simulink library "Testrig_4Post_Inputs"  (R2026a)
settings: Solver=VariableStepAuto
undefined symbols (not defined in the file or in its folder): Maneuver
libraries: dspsrcs4 x31, $bdroot x10, simulink x2
Description:
  | Testrig Inputs 4-Post Testrig
  | 
  | Copyright 2018-2024 The MathWorks, Inc.
settings Model: Creator=smiller  LastModifiedBy=andrei

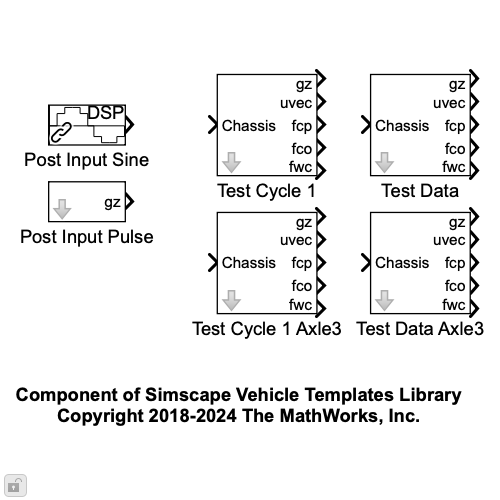
[thumbnail: Simulink's stored preview of the top-level diagram]
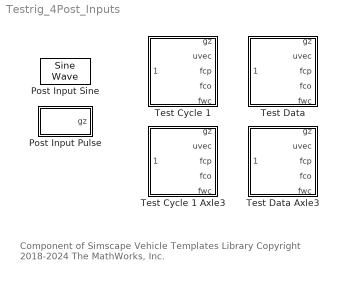
== system Testrig_4Post_Inputs ==
  note: Component of Simscape Vehicle Templates Library
      | Copyright 2018-2024 The MathWorks, Inc.
  Post Input Pulse : Subsystem  mask(Smooth Pulse){rise_time=0.1, pulse_length=2, wave_amplitude=5, wave_delay=1}
      mask prompts: rise_time "Rise/Fall Time (sec)"; pulse_length "Pulse Length (sec)"; wave_amplitude "Amplitude (m)"; wave_delay "Delay (sec)"
      mask help: Produces a pulse with a smooth start and finish, starting at a chosen time.
  Post Input Sine : dspsrcs4/Sine Wave  Amplitude=1  Frequency=100  Phase=0  SampleMode=Discrete  OutComplex=Real  CompMethod=Trigonometric fcn  TableSize=Speed  SampleTime=1/1000  SamplesPerFrame=1  ResetState=Restart at time zero  OutputFrames=off  dataType=double  wordLen=16  udDataType=sfix(16)  fracBitsMode=Best precision  numFracBits=15  OutDataTypeStr=double  LastOutDataTypeStr=double
  Test Cycle 1 : Subsystem  VariantControl=Test_Cycle_1  mask(Time-Based Post Height, Test Cycle 1, Four Posts){}
      mask help:
      | Sets road height beneath wheels to simulate a set of four tests: pitch, heave, roll, and bump.  The first three tests are sinusoidal, the last test is a trapezoid.
      |
      | This test is parameterized using the Maneuver data structure.  Use function sm_car_maneuverdata_testrig4Post_cycle1.m to create Maneuver and define this test.
  Test Cycle 1 Axle3 : Subsystem  mask(Time-Based Post Height, Test Cycle 1, 6 Posts){}
      mask help:
      | Sets road height beneath wheels to simulate a set of four tests: pitch, heave, roll, and bump.  The first three tests are sinusoidal, the last test is a trapezoid.
      |
      | This test is parameterized using the Maneuver data structure.  Use function sm_car_maneuverdata_testrig4Post_cycle1.m to create Maneuver and define this test.
  Test Data : Subsystem  VariantControl=Test_Cycle_1  mask(Time-Based Road Height, Four Post){table_postL1=Maneuver.PostL1.z.Value, brkpts_postL1=Maneuver.PostL1.t.Value, interp_postL1=Maneuver.PostL1.InterpMethod.Value, table_postR1=Maneuver.PostR1.z.Value, brkpts_postR1=Maneuver.PostR1.t.Value, interp_postR1=Maneuver.PostR1.InterpMethod.Value, table_postL2=Maneuver.PostL2.z.Value, brkpts_postL2=Maneuver.PostL2.t.Value, interp_postL2=Maneuver.PostL2.InterpMethod.Value, table_postR2=Maneuver.PostR2.z.Value, brkpts_postR2=Maneuver.PostR2.t.Value, interp_postR2=Maneuver.PostR2.InterpMethod.Value}
      mask prompts: table_postL1 "Height (m)"; brkpts_postL1 "Time (sec)"; interp_postL1 "Interpolation"; table_postR1 "Height (m)"; brkpts_postR1 "Time (sec)"; interp_postR1 "Interpolation"; table_postL2 "Height (m)"; brkpts_postL2 "Time (sec)"; interp_postL2 "Interpolation"; table_postR2 "Height (m)"; brkpts_postR2 "Time (sec)"; interp_postR2 "Interpolation"
      mask help: Sets road height based on simulation time. Used in postrig tests to control post based on generated or measured data. Set interpolation method to a string value that matches options for Lookup Table 1D block. Other outputs are held at their defaults.
      mask init:
      | bh = gcb;
      | set_param([bh '/Lookup Table L1'],'InterpMethod',interp_postL1);
      | set_param([bh '/Lookup Table R1'],'InterpMethod',interp_postR1);
      | set_param([bh '/Lookup Table L2'],'InterpMethod',interp_postL2);
      | set_param([bh '/Lookup Table R2'],'InterpMethod',interp_postR2);
      mask TypeOptions table_postL1: Lookup Table L1/Table
      mask TypeOptions brkpts_postL1: Lookup Table L1/BreakpointsForDimension1
      mask TypeOptions table_postR1: Lookup Table R1/Table
      mask TypeOptions brkpts_postR1: Lookup Table R1/BreakpointsForDimension1
      mask TypeOptions table_postL2: Lookup Table L2/Table
      mask TypeOptions brkpts_postL2: Lookup Table L2/BreakpointsForDimension1
      mask TypeOptions table_postR2: Lookup Table R2/Table
      mask TypeOptions brkpts_postR2: Lookup Table R2/BreakpointsForDimension1
      mask DialogControl cont_postL1 Prompt: Post L1 (Front Left)
      mask DialogControl cont_postR1 Prompt: Post R1 (Front Right)
      mask DialogControl cont_postL2 Prompt: Post L2 (Rear Left)
      mask DialogControl cont_postR2 Prompt: Post R2 (Rear Right)
  Test Data Axle3 : Subsystem  VariantControl=Test_Cycle_1  mask(Time-Based Road Height, Six Post Testrig){table_postL1=Maneuver.PostL1.z.Value, brkpts_postL1=Maneuver.PostL1.t.Value, interp_postL1=Maneuver.PostL1.InterpMethod.Value, table_postR1=Maneuver.PostR1.z.Value, brkpts_postR1=Maneuver.PostR1.t.Value, interp_postR1=Maneuver.PostR1.InterpMethod.Value, table_postL2=Maneuver.PostL2.z.Value, brkpts_postL2=Maneuver.PostL2.t.Value, interp_postL2=Maneuver.PostL2.InterpMethod.Value, table_postR2=Maneuver.PostR2.z.Value, brkpts_postR2=Maneuver.PostR2.t.Value, interp_postR2=Maneuver.PostR2.InterpMethod.Value, table_postL3=Maneuver.PostL3.z.Value, brkpts_postL3=Maneuver.PostL3.t.Value, interp_postL3=Maneuver.PostL3.InterpMethod.Value, table_postR3=Maneuver.PostR3.z.Value, brkpts_postR3=Maneuver.PostR3.t.Value, interp_postR3=Maneuver.PostR3.InterpMethod.Value}
      mask prompts: table_postL1 "Height (m)"; brkpts_postL1 "Time (sec)"; interp_postL1 "Interpolation"; table_postR1 "Height (m)"; brkpts_postR1 "Time (sec)"; interp_postR1 "Interpolation"; table_postL2 "Height (m)"; brkpts_postL2 "Time (sec)"; interp_postL2 "Interpolation"; table_postR2 "Height (m)"; brkpts_postR2 "Time (sec)"; interp_postR2 "Interpolation"; table_postL3 "Height (m)"; brkpts_postL3 "Time (sec)"; interp_postL3 "Interpolation"; table_postR3 "Height (m)"; brkpts_postR3 "Time (sec)"; interp_postR3 "Interpolation"
      mask help: Sets road height based on simulation time. Used in six-post testrigs to control post height based on generated or measured data. Set interpolation method to a string value that matches options for Lookup Table 1D block. Other outputs are held at their defaults.
      mask init:
      | bh = gcb;
      | set_param([bh '/Lookup Table L1'],'InterpMethod',interp_postL1);
      | set_param([bh '/Lookup Table R1'],'InterpMethod',interp_postR1);
      | set_param([bh '/Lookup Table L2'],'InterpMethod',interp_postL2);
      | set_param([bh '/Lookup Table R2'],'InterpMethod',interp_postR2);
      | set_param([bh '/Lookup Table L3'],'InterpMethod',interp_postL3);
      | set_param([bh '/Lookup Table R3'],'InterpMethod',interp_postR3);
      mask TypeOptions table_postL1: Lookup Table L1/Table
      mask TypeOptions brkpts_postL1: Lookup Table L1/BreakpointsForDimension1
      mask TypeOptions table_postR1: Lookup Table R1/Table
      mask TypeOptions brkpts_postR1: Lookup Table R1/BreakpointsForDimension1
      mask TypeOptions table_postL2: Lookup Table L2/Table
      mask TypeOptions brkpts_postL2: Lookup Table L2/BreakpointsForDimension1
      mask TypeOptions table_postR2: Lookup Table R2/Table
      mask TypeOptions brkpts_postR2: Lookup Table R2/BreakpointsForDimension1
      mask TypeOptions table_postL3: Lookup Table L3/Table
      mask TypeOptions brkpts_postL3: Lookup Table L3/BreakpointsForDimension1
      mask TypeOptions table_postR3: Lookup Table R3/Table
      mask TypeOptions brkpts_postR3: Lookup Table R3/BreakpointsForDimension1
      mask DialogControl cont_postL1 Prompt: Post L1 (Axle 1, Left)
      mask DialogControl cont_postR1 Prompt: Post R1 (Axle 1, Right)
      mask DialogControl cont_postL2 Prompt: Post L2 (Axle 2, Left)
      mask DialogControl cont_postR2 Prompt: Post R2 (Axle 2, Right)
      mask DialogControl cont_postL3 Prompt: Post L3  (Axle 3, Left)
      mask DialogControl cont_postR3 Prompt: Post R3  (Axle 3, Right)

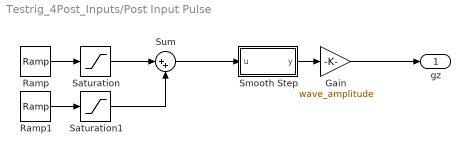
== system Testrig_4Post_Inputs/Post Input Pulse ==
  Gain : Gain  Gain=wave_amplitude
  Ramp : simulink/Sources/Ramp  slope=1/rise_time  start=wave_delay  InitialOutput=0
  Ramp1 : simulink/Sources/Ramp  slope=-1/rise_time  start=wave_delay+pulse_length-rise_time  InitialOutput=0
  Saturation : Saturate  UpperLimit=1  LowerLimit=0
  Saturation1 : Saturate  UpperLimit=0  LowerLimit=-1
  Smooth Step : Subsystem  mask(Smooth step function){step_start=0, step_finish=1, min_out=0, max_out=1}
      mask prompts: step_start "Start Step (u)"; step_finish "Finish Step (u)"; min_out "Minimum output (y)"; max_out "Maximum output (y)"
      mask help:
      | Smooth step function
      | y=3u^2-2u^3
      | Input and output ranges scaled by parameters.
  Sum : Sum  Inputs=|++
  gz : Outport  VectorParamsAs1DForOutWhenUnconnected=off
  wires:
  Gain/1 -> gz/1
  Ramp/1 -> Saturation/1
  Smooth Step/1(y) -> Gain/1
  Saturation/1 -> Sum/1
  Ramp1/1 -> Saturation1/1
  Saturation1/1 -> Sum/2
  Sum/1 -> Smooth Step/1(u)

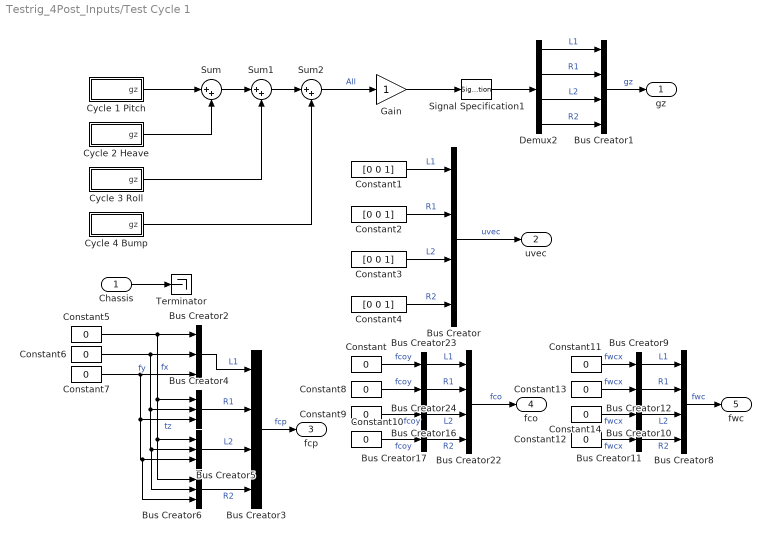
== system Testrig_4Post_Inputs/Test Cycle 1 ==
  Chassis : Inport
  Bus Creator{,1,3,8,22} (5 alike) : BusCreator  Inputs=4
  Bus Creator{9..12,16..17,23..24} (8 alike) : BusCreator  Inputs=1
  Bus Creator{2,4..6} (4 alike) : BusCreator  Inputs=3
  Constant{,5..14} (11 alike) : Constant  Value=0
  Constant{1..4} (4 alike) : Constant  Value=[0 0 1]
  Cycle 1 Pitch : Subsystem
  Cycle 2 Heave : Subsystem
  Cycle 3 Roll : Subsystem
  Cycle 4 Bump : Subsystem
  Demux2 : Demux
  Gain : Gain
  Signal Specification1 : SignalSpecification  Unit=m
  Sum : Sum  Inputs=|++
  Sum1 : Sum  Inputs=|++
  Sum2 : Sum  Inputs=|++
  Terminator : Terminator
  gz : Outport  VectorParamsAs1DForOutWhenUnconnected=off
  uvec : Outport  Port=2  VectorParamsAs1DForOutWhenUnconnected=off
  fcp : Outport  Port=3  VectorParamsAs1DForOutWhenUnconnected=off
  fco : Outport  Port=4  VectorParamsAs1DForOutWhenUnconnected=off
  fwc : Outport  Port=5  VectorParamsAs1DForOutWhenUnconnected=off
  wires:
  Constant7/1 -> Bus Creator2/3, Bus Creator4/3, Bus Creator5/3, Bus Creator6/3  "tz"
  Constant6/1 -> Bus Creator2/2, Bus Creator4/2, Bus Creator5/2, Bus Creator6/2  "fy"
  Constant5/1 -> Bus Creator2/1, Bus Creator4/1, Bus Creator5/1, Bus Creator6/1  "fx"
  Bus Creator6/1 -> Bus Creator3/4  "R2"
  Bus Creator5/1 -> Bus Creator3/3  "L2"
  Bus Creator2/1 -> Bus Creator3/1  "L1"
  Bus Creator4/1 -> Bus Creator3/2  "R1"
  Bus Creator3/1 -> fcp/1  "fcp"
  Cycle 2 Heave/1(gz) -> Sum/2
  Sum2/1 -> Gain/1  "All"
  Cycle 1 Pitch/1(gz) -> Sum/1
  Sum/1 -> Sum1/1
  Cycle 3 Roll/1(gz) -> Sum1/2
  Sum1/1 -> Sum2/1
  Cycle 4 Bump/1(gz) -> Sum2/2
  Gain/1 -> Signal Specification1/1
  Chassis/1 -> Terminator/1
  Constant4/1 -> Bus Creator/4  "R2"
  Bus Creator/1 -> uvec/1  "uvec"
  Constant1/1 -> Bus Creator/1  "L1"
  Constant2/1 -> Bus Creator/2  "R1"
  Constant3/1 -> Bus Creator/3  "L2"
  Signal Specification1/1 -> Demux2/1
  Demux2/3 -> Bus Creator1/3  "L2"
  Bus Creator1/1 -> gz/1  "gz"
  Demux2/4 -> Bus Creator1/4  "R2"
  Demux2/2 -> Bus Creator1/2  "R1"
  Demux2/1 -> Bus Creator1/1  "L1"
  Bus Creator12/1 -> Bus Creator8/2  "R1"
  Bus Creator24/1 -> Bus Creator22/2  "R1"
  Bus Creator10/1 -> Bus Creator8/3  "L2"
  Bus Creator9/1 -> Bus Creator8/1  "L1"
  Bus Creator16/1 -> Bus Creator22/3  "L2"
  Bus Creator22/1 -> fco/1  "fco"
  Bus Creator23/1 -> Bus Creator22/1  "L1"
  Bus Creator17/1 -> Bus Creator22/4  "R2"
  Constant8/1 -> Bus Creator24/1  "fcoy"
  Constant10/1 -> Bus Creator17/1  "fcoy"
  Constant9/1 -> Bus Creator16/1  "fcoy"
  Constant12/1 -> Bus Creator11/1  "fwcx"
  Constant14/1 -> Bus Creator10/1  "fwcx"
  Constant13/1 -> Bus Creator12/1  "fwcx"
  Bus Creator8/1 -> fwc/1  "fwc"
  Constant11/1 -> Bus Creator9/1  "fwcx"
  Constant/1 -> Bus Creator23/1  "fcoy"
  Bus Creator11/1 -> Bus Creator8/4  "R2"

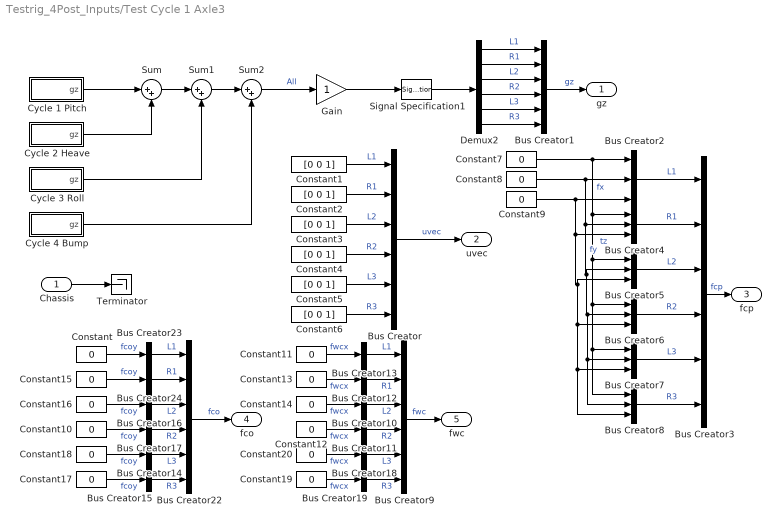
== system Testrig_4Post_Inputs/Test Cycle 1 Axle3 ==
  Chassis : Inport
  Bus Creator{,1,3,9,22} (5 alike) : BusCreator  Inputs=6
  Bus Creator{10..19,23..24} (12 alike) : BusCreator  Inputs=1
  Bus Creator{2,4..8} (6 alike) : BusCreator  Inputs=3
  Constant{,7..20} (15 alike) : Constant  Value=0
  Constant{1..6} (6 alike) : Constant  Value=[0 0 1]
  Cycle 1 Pitch : Subsystem
  Cycle 2 Heave : Subsystem
  Cycle 3 Roll : Subsystem
  Cycle 4 Bump : Subsystem
  Demux2 : Demux  Outputs=6
  Gain : Gain
  Signal Specification1 : SignalSpecification  Unit=m
  Sum : Sum  Inputs=|++
  Sum1 : Sum  Inputs=|++
  Sum2 : Sum  Inputs=|++
  Terminator : Terminator
  gz : Outport  VectorParamsAs1DForOutWhenUnconnected=off
  uvec : Outport  Port=2  VectorParamsAs1DForOutWhenUnconnected=off
  fcp : Outport  Port=3  VectorParamsAs1DForOutWhenUnconnected=off
  fco : Outport  Port=4  VectorParamsAs1DForOutWhenUnconnected=off
  fwc : Outport  Port=5  VectorParamsAs1DForOutWhenUnconnected=off
  wires:
  Demux2/1 -> Bus Creator1/1  "L1"
  Demux2/2 -> Bus Creator1/2  "R1"
  Demux2/4 -> Bus Creator1/4  "R2"
  Bus Creator1/1 -> gz/1  "gz"
  Demux2/3 -> Bus Creator1/3  "L2"
  Signal Specification1/1 -> Demux2/1
  Constant3/1 -> Bus Creator/3  "L2"
  Constant2/1 -> Bus Creator/2  "R1"
  Constant1/1 -> Bus Creator/1  "L1"
  Bus Creator/1 -> uvec/1  "uvec"
  Constant4/1 -> Bus Creator/4  "R2"
  Chassis/1 -> Terminator/1
  Gain/1 -> Signal Specification1/1
  Cycle 4 Bump/1(gz) -> Sum2/2
  Sum1/1 -> Sum2/1
  Cycle 3 Roll/1(gz) -> Sum1/2
  Sum/1 -> Sum1/1
  Cycle 1 Pitch/1(gz) -> Sum/1
  Sum2/1 -> Gain/1  "All"
  Cycle 2 Heave/1(gz) -> Sum/2
  Constant6/1 -> Bus Creator/6  "R3"
  Constant5/1 -> Bus Creator/5  "L3"
  Demux2/5 -> Bus Creator1/5  "L3"
  Demux2/6 -> Bus Creator1/6  "R3"
  Bus Creator6/1 -> Bus Creator3/4  "R2"
  Bus Creator4/1 -> Bus Creator3/2  "R1"
  Constant7/1 -> Bus Creator2/1, Bus Creator8/1, Bus Creator7/1, Bus Creator6/1, Bus Creator5/1, Bus Creator4/1  "fx"
  Bus Creator2/1 -> Bus Creator3/1  "L1"
  Bus Creator3/1 -> fcp/1  "fcp"
  Bus Creator5/1 -> Bus Creator3/3  "L2"
  Constant8/1 -> Bus Creator2/2, Bus Creator5/2, Bus Creator8/2, Bus Creator7/2, Bus Creator6/2, Bus Creator4/2  "fy"
  Constant9/1 -> Bus Creator2/3, Bus Creator5/3, Bus Creator6/3, Bus Creator8/3, Bus Creator7/3, Bus Creator4/3  "tz"
  Bus Creator7/1 -> Bus Creator3/5  "L3"
  Bus Creator8/1 -> Bus Creator3/6  "R3"
  Bus Creator12/1 -> Bus Creator9/2  "R1"
  Bus Creator24/1 -> Bus Creator22/2  "R1"
  Bus Creator10/1 -> Bus Creator9/3  "L2"
  Bus Creator13/1 -> Bus Creator9/1  "L1"
  Bus Creator16/1 -> Bus Creator22/3  "L2"
  Bus Creator22/1 -> fco/1  "fco"
  Bus Creator23/1 -> Bus Creator22/1  "L1"
  Bus Creator17/1 -> Bus Creator22/4  "R2"
  Constant15/1 -> Bus Creator24/1  "fcoy"
  Constant10/1 -> Bus Creator17/1  "fcoy"
  Constant16/1 -> Bus Creator16/1  "fcoy"
  Constant12/1 -> Bus Creator11/1  "fwcx"
  Constant14/1 -> Bus Creator10/1  "fwcx"
  Constant13/1 -> Bus Creator12/1  "fwcx"
  Bus Creator9/1 -> fwc/1  "fwc"
  Constant11/1 -> Bus Creator13/1  "fwcx"
  Constant/1 -> Bus Creator23/1  "fcoy"
  Bus Creator11/1 -> Bus Creator9/4  "R2"
  Constant18/1 -> Bus Creator14/1  "fcoy"
  Constant17/1 -> Bus Creator15/1  "fcoy"
  Bus Creator15/1 -> Bus Creator22/6  "R3"
  Bus Creator14/1 -> Bus Creator22/5  "L3"
  Bus Creator19/1 -> Bus Creator9/6  "R3"
  Constant20/1 -> Bus Creator18/1  "fwcx"
  Constant19/1 -> Bus Creator19/1  "fwcx"
  Bus Creator18/1 -> Bus Creator9/5  "L3"

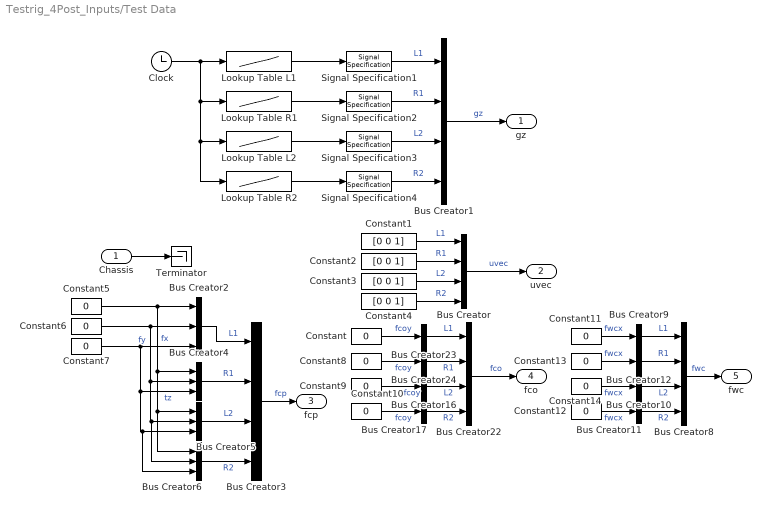
== system Testrig_4Post_Inputs/Test Data ==
  Chassis : Inport
  Bus Creator{,1,3,8,22} (5 alike) : BusCreator  Inputs=4
  Bus Creator{9..12,16..17,23..24} (8 alike) : BusCreator  Inputs=1
  Bus Creator{2,4..6} (4 alike) : BusCreator  Inputs=3
  Clock : Clock
  Constant{,5..14} (11 alike) : Constant  Value=0
  Constant{1..4} (4 alike) : Constant  Value=[0 0 1]
  Lookup Table L1 : Lookup_n-D  NumberOfTableDimensions=1  BreakpointsForDimension1=brkpts_postL1  Table=table_postL1  InternalRulePriority=Speed  RndMeth=Simplest
  Lookup Table L2 : Lookup_n-D  NumberOfTableDimensions=1  BreakpointsForDimension1=brkpts_postL2  Table=table_postL2  InterpMethod=Cubic spline  InternalRulePriority=Speed  RndMeth=Simplest
  Lookup Table R1 : Lookup_n-D  NumberOfTableDimensions=1  BreakpointsForDimension1=brkpts_postR1  Table=table_postR1  InterpMethod=Cubic spline  InternalRulePriority=Speed  RndMeth=Simplest
  Lookup Table R2 : Lookup_n-D  NumberOfTableDimensions=1  BreakpointsForDimension1=brkpts_postR2  Table=table_postR2  InterpMethod=Cubic spline  InternalRulePriority=Speed  RndMeth=Simplest
  Signal Specification{1..4} (4 alike) : SignalSpecification  Unit=m
  Terminator : Terminator
  gz : Outport  VectorParamsAs1DForOutWhenUnconnected=off
  uvec : Outport  Port=2  VectorParamsAs1DForOutWhenUnconnected=off
  fcp : Outport  Port=3  VectorParamsAs1DForOutWhenUnconnected=off
  fco : Outport  Port=4  VectorParamsAs1DForOutWhenUnconnected=off
  fwc : Outport  Port=5  VectorParamsAs1DForOutWhenUnconnected=off
  wires:
  Bus Creator11/1 -> Bus Creator8/4  "R2"
  Constant/1 -> Bus Creator23/1  "fcoy"
  Constant11/1 -> Bus Creator9/1  "fwcx"
  Bus Creator8/1 -> fwc/1  "fwc"
  Constant13/1 -> Bus Creator12/1  "fwcx"
  Constant14/1 -> Bus Creator10/1  "fwcx"
  Constant12/1 -> Bus Creator11/1  "fwcx"
  Constant9/1 -> Bus Creator16/1  "fcoy"
  Constant10/1 -> Bus Creator17/1  "fcoy"
  Constant8/1 -> Bus Creator24/1  "fcoy"
  Bus Creator17/1 -> Bus Creator22/4  "R2"
  Bus Creator23/1 -> Bus Creator22/1  "L1"
  Bus Creator22/1 -> fco/1  "fco"
  Bus Creator16/1 -> Bus Creator22/3  "L2"
  Bus Creator9/1 -> Bus Creator8/1  "L1"
  Bus Creator10/1 -> Bus Creator8/3  "L2"
  Bus Creator24/1 -> Bus Creator22/2  "R1"
  Bus Creator12/1 -> Bus Creator8/2  "R1"
  Constant3/1 -> Bus Creator/3  "L2"
  Constant2/1 -> Bus Creator/2  "R1"
  Constant1/1 -> Bus Creator/1  "L1"
  Bus Creator/1 -> uvec/1  "uvec"
  Constant4/1 -> Bus Creator/4  "R2"
  Chassis/1 -> Terminator/1
  Bus Creator3/1 -> fcp/1  "fcp"
  Bus Creator4/1 -> Bus Creator3/2  "R1"
  Bus Creator2/1 -> Bus Creator3/1  "L1"
  Bus Creator5/1 -> Bus Creator3/3  "L2"
  Bus Creator6/1 -> Bus Creator3/4  "R2"
  Constant5/1 -> Bus Creator6/1, Bus Creator5/1, Bus Creator4/1, Bus Creator2/1  "fx"
  Constant6/1 -> Bus Creator6/2, Bus Creator5/2, Bus Creator4/2, Bus Creator2/2  "fy"
  Constant7/1 -> Bus Creator6/3, Bus Creator5/3, Bus Creator4/3, Bus Creator2/3  "tz"
  Clock/1 -> Lookup Table L1/1, Lookup Table R2/1, Lookup Table L2/1, Lookup Table R1/1
  Lookup Table R2/1 -> Signal Specification4/1
  Bus Creator1/1 -> gz/1  "gz"
  Lookup Table L1/1 -> Signal Specification1/1
  Lookup Table L2/1 -> Signal Specification3/1
  Signal Specification3/1 -> Bus Creator1/3  "L2"
  Signal Specification2/1 -> Bus Creator1/2  "R1"
  Signal Specification1/1 -> Bus Creator1/1  "L1"
  Signal Specification4/1 -> Bus Creator1/4  "R2"
  Lookup Table R1/1 -> Signal Specification2/1

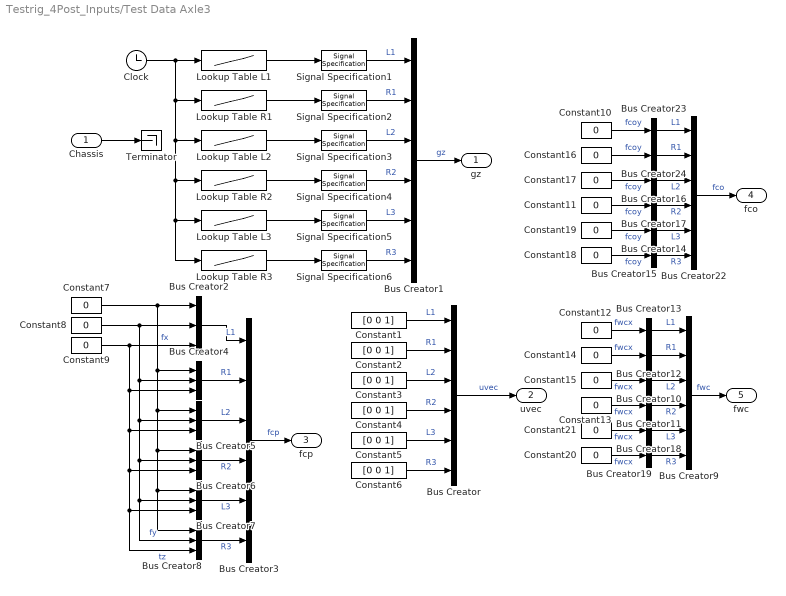
== system Testrig_4Post_Inputs/Test Data Axle3 ==
  Chassis : Inport
  Bus Creator{,1,3,9,22} (5 alike) : BusCreator  Inputs=6
  Bus Creator{10..19,23..24} (12 alike) : BusCreator  Inputs=1
  Bus Creator{2,4..8} (6 alike) : BusCreator  Inputs=3
  Clock : Clock
  Constant{1..6} (6 alike) : Constant  Value=[0 0 1]
  Constant{7..21} (15 alike) : Constant  Value=0
  Lookup Table L1 : Lookup_n-D  NumberOfTableDimensions=1  BreakpointsForDimension1=brkpts_postL1  Table=table_postL1  InternalRulePriority=Speed  RndMeth=Simplest
  Lookup Table L2 : Lookup_n-D  NumberOfTableDimensions=1  BreakpointsForDimension1=brkpts_postL2  Table=table_postL2  InterpMethod=Cubic spline  InternalRulePriority=Speed  RndMeth=Simplest
  Lookup Table L3 : Lookup_n-D  NumberOfTableDimensions=1  BreakpointsForDimension1=brkpts_postL3  Table=table_postL3  InterpMethod=Cubic spline  InternalRulePriority=Speed  RndMeth=Simplest
  Lookup Table R1 : Lookup_n-D  NumberOfTableDimensions=1  BreakpointsForDimension1=brkpts_postR1  Table=table_postR1  InterpMethod=Cubic spline  InternalRulePriority=Speed  RndMeth=Simplest
  Lookup Table R2 : Lookup_n-D  NumberOfTableDimensions=1  BreakpointsForDimension1=brkpts_postR2  Table=table_postR2  InterpMethod=Cubic spline  InternalRulePriority=Speed  RndMeth=Simplest
  Lookup Table R3 : Lookup_n-D  NumberOfTableDimensions=1  BreakpointsForDimension1=brkpts_postR3  Table=table_postR3  InterpMethod=Cubic spline  InternalRulePriority=Speed  RndMeth=Simplest
  Signal Specification{1..6} (6 alike) : SignalSpecification  Unit=m
  Terminator : Terminator
  gz : Outport  VectorParamsAs1DForOutWhenUnconnected=off
  uvec : Outport  Port=2  VectorParamsAs1DForOutWhenUnconnected=off
  fcp : Outport  Port=3  VectorParamsAs1DForOutWhenUnconnected=off
  fco : Outport  Port=4  VectorParamsAs1DForOutWhenUnconnected=off
  fwc : Outport  Port=5  VectorParamsAs1DForOutWhenUnconnected=off
  wires:
  Lookup Table R1/1 -> Signal Specification2/1
  Signal Specification4/1 -> Bus Creator1/4  "R2"
  Signal Specification1/1 -> Bus Creator1/1  "L1"
  Signal Specification2/1 -> Bus Creator1/2  "R1"
  Signal Specification3/1 -> Bus Creator1/3  "L2"
  Lookup Table L2/1 -> Signal Specification3/1
  Lookup Table L1/1 -> Signal Specification1/1
  Bus Creator1/1 -> gz/1  "gz"
  Lookup Table R2/1 -> Signal Specification4/1
  Chassis/1 -> Terminator/1
  Constant5/1 -> Bus Creator/5  "L3"
  Bus Creator2/1 -> Bus Creator3/1  "L1"
  Constant7/1 -> Bus Creator6/1, Bus Creator7/1, Bus Creator8/1, Bus Creator5/1, Bus Creator4/1, Bus Creator2/1  "fx"
  Constant6/1 -> Bus Creator/6  "R3"
  Bus Creator6/1 -> Bus Creator3/4  "R2"
  Constant18/1 -> Bus Creator15/1  "fcoy"
  Constant14/1 -> Bus Creator12/1  "fwcx"
  Bus Creator13/1 -> Bus Creator9/1  "L1"
  Constant17/1 -> Bus Creator16/1  "fcoy"
  Constant3/1 -> Bus Creator/3  "L2"
  Bus Creator19/1 -> Bus Creator9/6  "R3"
  Bus Creator4/1 -> Bus Creator3/2  "R1"
  Bus Creator22/1 -> fco/1  "fco"
  Bus Creator18/1 -> Bus Creator9/5  "L3"
  Bus Creator8/1 -> Bus Creator3/6  "R3"
  Bus Creator12/1 -> Bus Creator9/2  "R1"
  Constant2/1 -> Bus Creator/2  "R1"
  Bus Creator/1 -> uvec/1  "uvec"
  Bus Creator7/1 -> Bus Creator3/5  "L3"
  Constant4/1 -> Bus Creator/4  "R2"
  Bus Creator10/1 -> Bus Creator9/3  "L2"
  Constant11/1 -> Bus Creator17/1  "fcoy"
  Bus Creator14/1 -> Bus Creator22/5  "L3"
  Constant16/1 -> Bus Creator24/1  "fcoy"
  Constant12/1 -> Bus Creator13/1  "fwcx"
  Constant21/1 -> Bus Creator18/1  "fwcx"
  Constant1/1 -> Bus Creator/1  "L1"
  Constant10/1 -> Bus Creator23/1  "fcoy"
  Bus Creator11/1 -> Bus Creator9/4  "R2"
  Bus Creator23/1 -> Bus Creator22/1  "L1"
  Constant9/1 -> Bus Creator8/3, Bus Creator7/3, Bus Creator6/3, Bus Creator5/3, Bus Creator4/3, Bus Creator2/3  "tz"
  Bus Creator5/1 -> Bus Creator3/3  "L2"
  Constant15/1 -> Bus Creator10/1  "fwcx"
  Bus Creator15/1 -> Bus Creator22/6  "R3"
  Constant19/1 -> Bus Creator14/1  "fcoy"
  Constant13/1 -> Bus Creator11/1  "fwcx"
  Bus Creator3/1 -> fcp/1  "fcp"
  Bus Creator24/1 -> Bus Creator22/2  "R1"
  Constant8/1 -> Bus Creator8/2, Bus Creator7/2, Bus Creator6/2, Bus Creator5/2, Bus Creator4/2, Bus Creator2/2  "fy"
  Bus Creator16/1 -> Bus Creator22/3  "L2"
  Bus Creator17/1 -> Bus Creator22/4  "R2"
  Bus Creator9/1 -> fwc/1  "fwc"
  Constant20/1 -> Bus Creator19/1  "fwcx"
  Clock/1 -> Lookup Table R1/1, Lookup Table L2/1, Lookup Table R3/1, Lookup Table L3/1, Lookup Table R2/1, Lookup Table L1/1
  Lookup Table R3/1 -> Signal Specification6/1
  Lookup Table L3/1 -> Signal Specification5/1
  Signal Specification5/1 -> Bus Creator1/5  "L3"
  Signal Specification6/1 -> Bus Creator1/6  "R3"

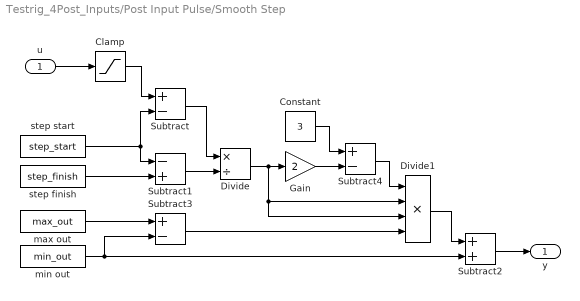
== system Testrig_4Post_Inputs/Post Input Pulse/Smooth Step ==
  u : Inport
  Clamp : Saturate  UpperLimit=step_finish  LowerLimit=step_start
  Constant : Constant  Value=3
  Divide : Product  Inputs=*/
  Divide1 : Product  Inputs=****
  Gain : Gain  Gain=2
  Subtract : Sum  Inputs=+-
  Subtract1 : Sum  Inputs=-+
  Subtract2 : Sum
  Subtract3 : Sum  Inputs=+-
  Subtract4 : Sum  Inputs=+-
  max out : Constant  Value=max_out
  min out : Constant  Value=min_out
  step finish : Constant  Value=step_finish
  step start : Constant  Value=step_start
  y : Outport  VectorParamsAs1DForOutWhenUnconnected=off
  wires:
  step start/1 -> Subtract1/1, Subtract/2
  u/1 -> Clamp/1
  Subtract1/1 -> Divide/2
  Divide/1 -> Gain/1, Divide1/2, Divide1/3
  Subtract/1 -> Divide/1
  Subtract2/1 -> y/1
  Constant/1 -> Subtract4/1
  min out/1 -> Subtract2/2, Subtract3/2
  max out/1 -> Subtract3/1
  Clamp/1 -> Subtract/1
  step finish/1 -> Subtract1/2
  Divide1/1 -> Subtract2/1
  Gain/1 -> Subtract4/2
  Subtract4/1 -> Divide1/1
  Subtract3/1 -> Divide1/4

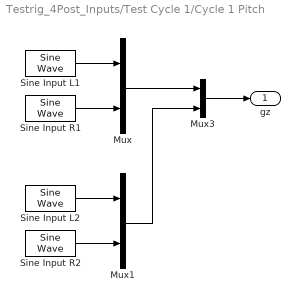
== system Testrig_4Post_Inputs/Test Cycle 1/Cycle 1 Pitch ==
  Mux : Mux  Inputs=2
  Mux1 : Mux  Inputs=2
  Mux3 : Mux  Inputs=2
  Sine Input L1 : dspsrcs4/Sine Wave  Amplitude=1  Frequency=100  Phase=0  SampleMode=Discrete  OutComplex=Real  CompMethod=Trigonometric fcn  TableSize=Speed  SampleTime=1/1000  SamplesPerFrame=1  ResetState=Restart at time zero  OutputFrames=off  dataType=double  wordLen=16  udDataType=sfix(16)  fracBitsMode=Best precision  numFracBits=15  OutDataTypeStr=double  LastOutDataTypeStr=double
  Sine Input L2 : dspsrcs4/Sine Wave  Amplitude=1  Frequency=100  Phase=0  SampleMode=Discrete  OutComplex=Real  CompMethod=Trigonometric fcn  TableSize=Speed  SampleTime=1/1000  SamplesPerFrame=1  ResetState=Restart at time zero  OutputFrames=off  dataType=double  wordLen=16  udDataType=sfix(16)  fracBitsMode=Best precision  numFracBits=15  OutDataTypeStr=double  LastOutDataTypeStr=double
  Sine Input R1 : dspsrcs4/Sine Wave  Amplitude=1  Frequency=100  Phase=0  SampleMode=Discrete  OutComplex=Real  CompMethod=Trigonometric fcn  TableSize=Speed  SampleTime=1/1000  SamplesPerFrame=1  ResetState=Restart at time zero  OutputFrames=off  dataType=double  wordLen=16  udDataType=sfix(16)  fracBitsMode=Best precision  numFracBits=15  OutDataTypeStr=double  LastOutDataTypeStr=double
  Sine Input R2 : dspsrcs4/Sine Wave  Amplitude=1  Frequency=100  Phase=0  SampleMode=Discrete  OutComplex=Real  CompMethod=Trigonometric fcn  TableSize=Speed  SampleTime=1/1000  SamplesPerFrame=1  ResetState=Restart at time zero  OutputFrames=off  dataType=double  wordLen=16  udDataType=sfix(16)  fracBitsMode=Best precision  numFracBits=15  OutDataTypeStr=double  LastOutDataTypeStr=double
  gz : Outport  VectorParamsAs1DForOutWhenUnconnected=off
  wires:
  Sine Input L1/1 -> Mux/1
  Sine Input R1/1 -> Mux/2
  Mux/1 -> Mux3/1
  Mux3/1 -> gz/1
  Mux1/1 -> Mux3/2
  Sine Input R2/1 -> Mux1/2
  Sine Input L2/1 -> Mux1/1

== system Testrig_4Post_Inputs/Test Cycle 1/Cycle 2 Heave ==
  Mux : Mux  Inputs=2
  Mux1 : Mux  Inputs=2
  Mux3 : Mux  Inputs=2
  Sine Input L1 : dspsrcs4/Sine Wave  Amplitude=1  Frequency=100  Phase=0  SampleMode=Discrete  OutComplex=Real  CompMethod=Trigonometric fcn  TableSize=Speed  SampleTime=1/1000  SamplesPerFrame=1  ResetState=Restart at time zero  OutputFrames=off  dataType=double  wordLen=16  udDataType=sfix(16)  fracBitsMode=Best precision  numFracBits=15  OutDataTypeStr=double  LastOutDataTypeStr=double
  Sine Input L2 : dspsrcs4/Sine Wave  Amplitude=1  Frequency=100  Phase=0  SampleMode=Discrete  OutComplex=Real  CompMethod=Trigonometric fcn  TableSize=Speed  SampleTime=1/1000  SamplesPerFrame=1  ResetState=Restart at time zero  OutputFrames=off  dataType=double  wordLen=16  udDataType=sfix(16)  fracBitsMode=Best precision  numFracBits=15  OutDataTypeStr=double  LastOutDataTypeStr=double
  Sine Input R1 : dspsrcs4/Sine Wave  Amplitude=1  Frequency=100  Phase=0  SampleMode=Discrete  OutComplex=Real  CompMethod=Trigonometric fcn  TableSize=Speed  SampleTime=1/1000  SamplesPerFrame=1  ResetState=Restart at time zero  OutputFrames=off  dataType=double  wordLen=16  udDataType=sfix(16)  fracBitsMode=Best precision  numFracBits=15  OutDataTypeStr=double  LastOutDataTypeStr=double
  Sine Input R2 : dspsrcs4/Sine Wave  Amplitude=1  Frequency=100  Phase=0  SampleMode=Discrete  OutComplex=Real  CompMethod=Trigonometric fcn  TableSize=Speed  SampleTime=1/1000  SamplesPerFrame=1  ResetState=Restart at time zero  OutputFrames=off  dataType=double  wordLen=16  udDataType=sfix(16)  fracBitsMode=Best precision  numFracBits=15  OutDataTypeStr=double  LastOutDataTypeStr=double
  gz : Outport  VectorParamsAs1DForOutWhenUnconnected=off
  wires:
  Sine Input L2/1 -> Mux1/1
  Sine Input R2/1 -> Mux1/2
  Mux1/1 -> Mux3/2
  Mux3/1 -> gz/1
  Mux/1 -> Mux3/1
  Sine Input R1/1 -> Mux/2
  Sine Input L1/1 -> Mux/1

== system Testrig_4Post_Inputs/Test Cycle 1/Cycle 3 Roll ==
  Mux : Mux  Inputs=2
  Mux1 : Mux  Inputs=2
  Mux3 : Mux  Inputs=2
  Sine Input L1 : dspsrcs4/Sine Wave  Amplitude=1  Frequency=100  Phase=0  SampleMode=Discrete  OutComplex=Real  CompMethod=Trigonometric fcn  TableSize=Speed  SampleTime=1/1000  SamplesPerFrame=1  ResetState=Restart at time zero  OutputFrames=off  dataType=double  wordLen=16  udDataType=sfix(16)  fracBitsMode=Best precision  numFracBits=15  OutDataTypeStr=double  LastOutDataTypeStr=double
  Sine Input L2 : dspsrcs4/Sine Wave  Amplitude=1  Frequency=100  Phase=0  SampleMode=Discrete  OutComplex=Real  CompMethod=Trigonometric fcn  TableSize=Speed  SampleTime=1/1000  SamplesPerFrame=1  ResetState=Restart at time zero  OutputFrames=off  dataType=double  wordLen=16  udDataType=sfix(16)  fracBitsMode=Best precision  numFracBits=15  OutDataTypeStr=double  LastOutDataTypeStr=double
  Sine Input R1 : dspsrcs4/Sine Wave  Amplitude=1  Frequency=100  Phase=0  SampleMode=Discrete  OutComplex=Real  CompMethod=Trigonometric fcn  TableSize=Speed  SampleTime=1/1000  SamplesPerFrame=1  ResetState=Restart at time zero  OutputFrames=off  dataType=double  wordLen=16  udDataType=sfix(16)  fracBitsMode=Best precision  numFracBits=15  OutDataTypeStr=double  LastOutDataTypeStr=double
  Sine Input R2 : dspsrcs4/Sine Wave  Amplitude=1  Frequency=100  Phase=0  SampleMode=Discrete  OutComplex=Real  CompMethod=Trigonometric fcn  TableSize=Speed  SampleTime=1/1000  SamplesPerFrame=1  ResetState=Restart at time zero  OutputFrames=off  dataType=double  wordLen=16  udDataType=sfix(16)  fracBitsMode=Best precision  numFracBits=15  OutDataTypeStr=double  LastOutDataTypeStr=double
  gz : Outport  VectorParamsAs1DForOutWhenUnconnected=off
  wires:
  Sine Input L1/1 -> Mux/1
  Sine Input R1/1 -> Mux/2
  Mux/1 -> Mux3/1
  Mux3/1 -> gz/1
  Mux1/1 -> Mux3/2
  Sine Input R2/1 -> Mux1/2
  Sine Input L2/1 -> Mux1/1

== system Testrig_4Post_Inputs/Test Cycle 1/Cycle 4 Bump ==
  Mux : Mux  Inputs=2
  Mux2 : Mux  Inputs=2
  Mux3 : Mux  Inputs=2
  Pulse Input L1 : $bdroot/Post Input Pulse  rise_time=Maneuver.Bump.L1.tRise.Value  pulse_length=Maneuver.Bump.L1.tDuration.Value  wave_amplitude=Maneuver.Bump.L1.xAmplitude.Value  wave_delay=Maneuver.Bump.L1.tStart.Value
  Pulse Input L2 : $bdroot/Post Input Pulse  rise_time=Maneuver.Bump.L2.tRise.Value  pulse_length=Maneuver.Bump.L2.tDuration.Value  wave_amplitude=Maneuver.Bump.L2.xAmplitude.Value  wave_delay=Maneuver.Bump.L2.tStart.Value
  Pulse Input R1 : $bdroot/Post Input Pulse  rise_time=Maneuver.Bump.R1.tRise.Value  pulse_length=Maneuver.Bump.R1.tDuration.Value  wave_amplitude=Maneuver.Bump.R1.xAmplitude.Value  wave_delay=Maneuver.Bump.R1.tStart.Value
  Pulse Input R2 : $bdroot/Post Input Pulse  rise_time=Maneuver.Bump.R2.tRise.Value  pulse_length=Maneuver.Bump.R2.tDuration.Value  wave_amplitude=Maneuver.Bump.R2.xAmplitude.Value  wave_delay=Maneuver.Bump.R2.tStart.Value
  gz : Outport  VectorParamsAs1DForOutWhenUnconnected=off
  wires:
  Mux2/1 -> Mux3/2
  Mux3/1 -> gz/1
  Mux/1 -> Mux3/1
  Pulse Input R2/1 -> Mux2/2
  Pulse Input R1/1 -> Mux/2
  Pulse Input L1/1 -> Mux/1
  Pulse Input L2/1 -> Mux2/1

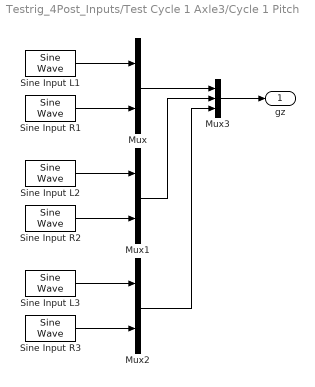
== system Testrig_4Post_Inputs/Test Cycle 1 Axle3/Cycle 1 Pitch ==
  Mux : Mux  Inputs=2
  Mux1 : Mux  Inputs=2
  Mux2 : Mux  Inputs=2
  Mux3 : Mux  Inputs=3
  Sine Input L1 : dspsrcs4/Sine Wave  Amplitude=1  Frequency=100  Phase=0  SampleMode=Discrete  OutComplex=Real  CompMethod=Trigonometric fcn  TableSize=Speed  SampleTime=1/1000  SamplesPerFrame=1  ResetState=Restart at time zero  OutputFrames=off  dataType=double  wordLen=16  udDataType=sfix(16)  fracBitsMode=Best precision  numFracBits=15  OutDataTypeStr=double  LastOutDataTypeStr=double
  Sine Input L2 : dspsrcs4/Sine Wave  Amplitude=1  Frequency=100  Phase=0  SampleMode=Discrete  OutComplex=Real  CompMethod=Trigonometric fcn  TableSize=Speed  SampleTime=1/1000  SamplesPerFrame=1  ResetState=Restart at time zero  OutputFrames=off  dataType=double  wordLen=16  udDataType=sfix(16)  fracBitsMode=Best precision  numFracBits=15  OutDataTypeStr=double  LastOutDataTypeStr=double
  Sine Input L3 : dspsrcs4/Sine Wave  Amplitude=1  Frequency=100  Phase=0  SampleMode=Discrete  OutComplex=Real  CompMethod=Trigonometric fcn  TableSize=Speed  SampleTime=1/1000  SamplesPerFrame=1  ResetState=Restart at time zero  OutputFrames=off  dataType=double  wordLen=16  udDataType=sfix(16)  fracBitsMode=Best precision  numFracBits=15  OutDataTypeStr=double  LastOutDataTypeStr=double
  Sine Input R1 : dspsrcs4/Sine Wave  Amplitude=1  Frequency=100  Phase=0  SampleMode=Discrete  OutComplex=Real  CompMethod=Trigonometric fcn  TableSize=Speed  SampleTime=1/1000  SamplesPerFrame=1  ResetState=Restart at time zero  OutputFrames=off  dataType=double  wordLen=16  udDataType=sfix(16)  fracBitsMode=Best precision  numFracBits=15  OutDataTypeStr=double  LastOutDataTypeStr=double
  Sine Input R2 : dspsrcs4/Sine Wave  Amplitude=1  Frequency=100  Phase=0  SampleMode=Discrete  OutComplex=Real  CompMethod=Trigonometric fcn  TableSize=Speed  SampleTime=1/1000  SamplesPerFrame=1  ResetState=Restart at time zero  OutputFrames=off  dataType=double  wordLen=16  udDataType=sfix(16)  fracBitsMode=Best precision  numFracBits=15  OutDataTypeStr=double  LastOutDataTypeStr=double
  Sine Input R3 : dspsrcs4/Sine Wave  Amplitude=1  Frequency=100  Phase=0  SampleMode=Discrete  OutComplex=Real  CompMethod=Trigonometric fcn  TableSize=Speed  SampleTime=1/1000  SamplesPerFrame=1  ResetState=Restart at time zero  OutputFrames=off  dataType=double  wordLen=16  udDataType=sfix(16)  fracBitsMode=Best precision  numFracBits=15  OutDataTypeStr=double  LastOutDataTypeStr=double
  gz : Outport  VectorParamsAs1DForOutWhenUnconnected=off
  wires:
  Sine Input L2/1 -> Mux1/1
  Sine Input R2/1 -> Mux1/2
  Mux1/1 -> Mux3/2
  Mux3/1 -> gz/1
  Mux/1 -> Mux3/1
  Sine Input R1/1 -> Mux/2
  Sine Input L1/1 -> Mux/1
  Mux2/1 -> Mux3/3
  Sine Input R3/1 -> Mux2/2
  Sine Input L3/1 -> Mux2/1

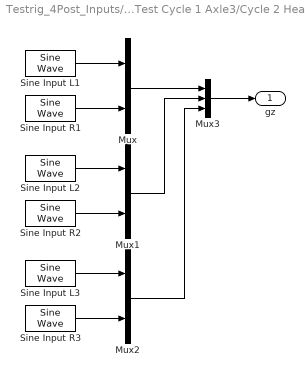
== system Testrig_4Post_Inputs/Test Cycle 1 Axle3/Cycle 2 Heave ==
  Mux : Mux  Inputs=2
  Mux1 : Mux  Inputs=2
  Mux2 : Mux  Inputs=2
  Mux3 : Mux  Inputs=3
  Sine Input L1 : dspsrcs4/Sine Wave  Amplitude=1  Frequency=100  Phase=0  SampleMode=Discrete  OutComplex=Real  CompMethod=Trigonometric fcn  TableSize=Speed  SampleTime=1/1000  SamplesPerFrame=1  ResetState=Restart at time zero  OutputFrames=off  dataType=double  wordLen=16  udDataType=sfix(16)  fracBitsMode=Best precision  numFracBits=15  OutDataTypeStr=double  LastOutDataTypeStr=double
  Sine Input L2 : dspsrcs4/Sine Wave  Amplitude=1  Frequency=100  Phase=0  SampleMode=Discrete  OutComplex=Real  CompMethod=Trigonometric fcn  TableSize=Speed  SampleTime=1/1000  SamplesPerFrame=1  ResetState=Restart at time zero  OutputFrames=off  dataType=double  wordLen=16  udDataType=sfix(16)  fracBitsMode=Best precision  numFracBits=15  OutDataTypeStr=double  LastOutDataTypeStr=double
  Sine Input L3 : dspsrcs4/Sine Wave  Amplitude=1  Frequency=100  Phase=0  SampleMode=Discrete  OutComplex=Real  CompMethod=Trigonometric fcn  TableSize=Speed  SampleTime=1/1000  SamplesPerFrame=1  ResetState=Restart at time zero  OutputFrames=off  dataType=double  wordLen=16  udDataType=sfix(16)  fracBitsMode=Best precision  numFracBits=15  OutDataTypeStr=double  LastOutDataTypeStr=double
  Sine Input R1 : dspsrcs4/Sine Wave  Amplitude=1  Frequency=100  Phase=0  SampleMode=Discrete  OutComplex=Real  CompMethod=Trigonometric fcn  TableSize=Speed  SampleTime=1/1000  SamplesPerFrame=1  ResetState=Restart at time zero  OutputFrames=off  dataType=double  wordLen=16  udDataType=sfix(16)  fracBitsMode=Best precision  numFracBits=15  OutDataTypeStr=double  LastOutDataTypeStr=double
  Sine Input R2 : dspsrcs4/Sine Wave  Amplitude=1  Frequency=100  Phase=0  SampleMode=Discrete  OutComplex=Real  CompMethod=Trigonometric fcn  TableSize=Speed  SampleTime=1/1000  SamplesPerFrame=1  ResetState=Restart at time zero  OutputFrames=off  dataType=double  wordLen=16  udDataType=sfix(16)  fracBitsMode=Best precision  numFracBits=15  OutDataTypeStr=double  LastOutDataTypeStr=double
  Sine Input R3 : dspsrcs4/Sine Wave  Amplitude=1  Frequency=100  Phase=0  SampleMode=Discrete  OutComplex=Real  CompMethod=Trigonometric fcn  TableSize=Speed  SampleTime=1/1000  SamplesPerFrame=1  ResetState=Restart at time zero  OutputFrames=off  dataType=double  wordLen=16  udDataType=sfix(16)  fracBitsMode=Best precision  numFracBits=15  OutDataTypeStr=double  LastOutDataTypeStr=double
  gz : Outport  VectorParamsAs1DForOutWhenUnconnected=off
  wires:
  Sine Input L1/1 -> Mux/1
  Sine Input R1/1 -> Mux/2
  Mux/1 -> Mux3/1
  Mux3/1 -> gz/1
  Mux1/1 -> Mux3/2
  Sine Input R2/1 -> Mux1/2
  Sine Input L2/1 -> Mux1/1
  Sine Input L3/1 -> Mux2/1
  Sine Input R3/1 -> Mux2/2
  Mux2/1 -> Mux3/3

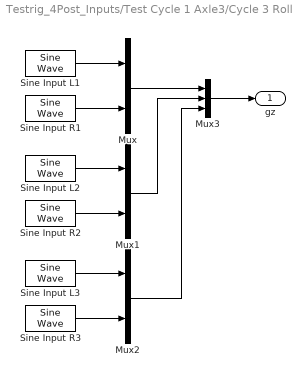
== system Testrig_4Post_Inputs/Test Cycle 1 Axle3/Cycle 3 Roll ==
  Mux : Mux  Inputs=2
  Mux1 : Mux  Inputs=2
  Mux2 : Mux  Inputs=2
  Mux3 : Mux  Inputs=3
  Sine Input L1 : dspsrcs4/Sine Wave  Amplitude=1  Frequency=100  Phase=0  SampleMode=Discrete  OutComplex=Real  CompMethod=Trigonometric fcn  TableSize=Speed  SampleTime=1/1000  SamplesPerFrame=1  ResetState=Restart at time zero  OutputFrames=off  dataType=double  wordLen=16  udDataType=sfix(16)  fracBitsMode=Best precision  numFracBits=15  OutDataTypeStr=double  LastOutDataTypeStr=double
  Sine Input L2 : dspsrcs4/Sine Wave  Amplitude=1  Frequency=100  Phase=0  SampleMode=Discrete  OutComplex=Real  CompMethod=Trigonometric fcn  TableSize=Speed  SampleTime=1/1000  SamplesPerFrame=1  ResetState=Restart at time zero  OutputFrames=off  dataType=double  wordLen=16  udDataType=sfix(16)  fracBitsMode=Best precision  numFracBits=15  OutDataTypeStr=double  LastOutDataTypeStr=double
  Sine Input L3 : dspsrcs4/Sine Wave  Amplitude=1  Frequency=100  Phase=0  SampleMode=Discrete  OutComplex=Real  CompMethod=Trigonometric fcn  TableSize=Speed  SampleTime=1/1000  SamplesPerFrame=1  ResetState=Restart at time zero  OutputFrames=off  dataType=double  wordLen=16  udDataType=sfix(16)  fracBitsMode=Best precision  numFracBits=15  OutDataTypeStr=double  LastOutDataTypeStr=double
  Sine Input R1 : dspsrcs4/Sine Wave  Amplitude=1  Frequency=100  Phase=0  SampleMode=Discrete  OutComplex=Real  CompMethod=Trigonometric fcn  TableSize=Speed  SampleTime=1/1000  SamplesPerFrame=1  ResetState=Restart at time zero  OutputFrames=off  dataType=double  wordLen=16  udDataType=sfix(16)  fracBitsMode=Best precision  numFracBits=15  OutDataTypeStr=double  LastOutDataTypeStr=double
  Sine Input R2 : dspsrcs4/Sine Wave  Amplitude=1  Frequency=100  Phase=0  SampleMode=Discrete  OutComplex=Real  CompMethod=Trigonometric fcn  TableSize=Speed  SampleTime=1/1000  SamplesPerFrame=1  ResetState=Restart at time zero  OutputFrames=off  dataType=double  wordLen=16  udDataType=sfix(16)  fracBitsMode=Best precision  numFracBits=15  OutDataTypeStr=double  LastOutDataTypeStr=double
  Sine Input R3 : dspsrcs4/Sine Wave  Amplitude=1  Frequency=100  Phase=0  SampleMode=Discrete  OutComplex=Real  CompMethod=Trigonometric fcn  TableSize=Speed  SampleTime=1/1000  SamplesPerFrame=1  ResetState=Restart at time zero  OutputFrames=off  dataType=double  wordLen=16  udDataType=sfix(16)  fracBitsMode=Best precision  numFracBits=15  OutDataTypeStr=double  LastOutDataTypeStr=double
  gz : Outport  VectorParamsAs1DForOutWhenUnconnected=off
  wires:
  Sine Input L2/1 -> Mux1/1
  Sine Input R2/1 -> Mux1/2
  Mux1/1 -> Mux3/2
  Mux3/1 -> gz/1
  Mux/1 -> Mux3/1
  Sine Input R1/1 -> Mux/2
  Sine Input L1/1 -> Mux/1
  Mux2/1 -> Mux3/3
  Sine Input R3/1 -> Mux2/2
  Sine Input L3/1 -> Mux2/1

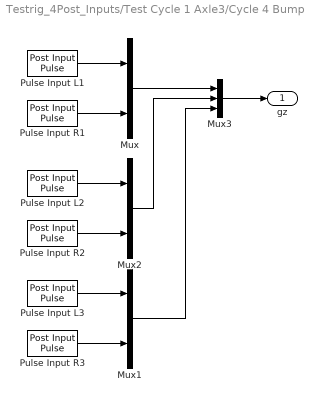
== system Testrig_4Post_Inputs/Test Cycle 1 Axle3/Cycle 4 Bump ==
  Mux : Mux  Inputs=2
  Mux1 : Mux  Inputs=2
  Mux2 : Mux  Inputs=2
  Mux3 : Mux  Inputs=3
  Pulse Input L1 : $bdroot/Post Input Pulse  rise_time=Maneuver.Bump.L1.tRise.Value  pulse_length=Maneuver.Bump.L1.tDuration.Value  wave_amplitude=Maneuver.Bump.L1.xAmplitude.Value  wave_delay=Maneuver.Bump.L1.tStart.Value
  Pulse Input L2 : $bdroot/Post Input Pulse  rise_time=Maneuver.Bump.L2.tRise.Value  pulse_length=Maneuver.Bump.L2.tDuration.Value  wave_amplitude=Maneuver.Bump.L2.xAmplitude.Value  wave_delay=Maneuver.Bump.L2.tStart.Value
  Pulse Input L3 : $bdroot/Post Input Pulse  rise_time=Maneuver.Bump.L3.tRise.Value  pulse_length=Maneuver.Bump.L3.tDuration.Value  wave_amplitude=Maneuver.Bump.L3.xAmplitude.Value  wave_delay=Maneuver.Bump.L3.tStart.Value
  Pulse Input R1 : $bdroot/Post Input Pulse  rise_time=Maneuver.Bump.R1.tRise.Value  pulse_length=Maneuver.Bump.R1.tDuration.Value  wave_amplitude=Maneuver.Bump.R1.xAmplitude.Value  wave_delay=Maneuver.Bump.R1.tStart.Value
  Pulse Input R2 : $bdroot/Post Input Pulse  rise_time=Maneuver.Bump.R2.tRise.Value  pulse_length=Maneuver.Bump.R2.tDuration.Value  wave_amplitude=Maneuver.Bump.R2.xAmplitude.Value  wave_delay=Maneuver.Bump.R2.tStart.Value
  Pulse Input R3 : $bdroot/Post Input Pulse  rise_time=Maneuver.Bump.R3.tRise.Value  pulse_length=Maneuver.Bump.R3.tDuration.Value  wave_amplitude=Maneuver.Bump.R3.xAmplitude.Value  wave_delay=Maneuver.Bump.R3.tStart.Value
  gz : Outport  VectorParamsAs1DForOutWhenUnconnected=off
  wires:
  Mux3/1 -> gz/1
  Pulse Input L1/1 -> Mux/1
  Mux2/1 -> Mux3/2
  Pulse Input L2/1 -> Mux2/1
  Pulse Input R1/1 -> Mux/2
  Pulse Input R2/1 -> Mux2/2
  Mux/1 -> Mux3/1
  Pulse Input R3/1 -> Mux1/2
  Pulse Input L3/1 -> Mux1/1
  Mux1/1 -> Mux3/3
